simulink model "GroundSourceHX_oldGfunction"  (R2018b)
settings: Solver=ode23t  StartTime=0.0  StopTime=7*24*3600  RelTol=1e-3
values from neighbouring files (symbols this model uses):
  Ad = zeros(DimAxi/2,DimAxi/2)    [parameter_CARNOTews.m]
  Ad0 = zeros(DimAxi/2,DimAxi/2)    [parameter_CARNOTews.m]
  Ar = a    [parameter_CARNOTews.m]
  Au = zeros(DimAxi/2,DimAxi/2)    [parameter_CARNOTews.m]
  Au0 = zeros(DimAxi/2,DimAxi/2)    [parameter_CARNOTews.m]
  Bd = zeros(DimAxi/2,DimAxi/2+1)    [parameter_CARNOTews.m]
  Bd0 = zeros(DimAxi/2,DimAxi/2+1)    [parameter_CARNOTews.m]
  Br = b    (= 0.718333333333)    [parameter_CARNOTews.m]
  Bu = zeros(DimAxi/2,DimAxi/2+1)    [parameter_CARNOTews.m]
  Bu0 = zeros(DimAxi/2,DimAxi/2+1)    [parameter_CARNOTews.m]
  c1 = zeros(DimAxi/2,Dim1)    [parameter_CARNOTews.m]
  c33 = zeros(DimAxi,DimAxi/2)    [parameter_CARNOTews.m]
  c4 = c41    [parameter_CARNOTews.m]
  Cd = eye(DimAxi/2)    [parameter_CARNOTews.m]
  Cdl = Cdl'    [parameter_CARNOTews.m]
  Cr = eye((DimRad-2)*DimAxi/2)    [parameter_CARNOTews.m]
  Cu = Cd    [parameter_CARNOTews.m]
  Dd = zeros(DimAxi/2,DimAxi/2+1)    [parameter_CARNOTews.m]
  Dl = Sondelaenge/DimAxi*2    (= 50)    [parameter_CARNOTews.m]
  Dr = zeros((DimRad-2)*DimAxi/2,DimAxi)    [parameter_CARNOTews.m]
  Du = zeros(DimAxi/2,DimAxi/2+1)    [parameter_CARNOTews.m]
  gfunction = zeros(length(t_Trichter),length(r_Trichter))    [parameter_CARNOTews.m]
  L1 = 1/R1    [parameter_CARNOTews.m]
  Rechenradius = rm    (= 5)    [parameter_CARNOTews.m]
  T_null = TEarth0(end,:)'    [parameter_CARNOTews.m]
  t_start = 50*8560*3600    (= 1540800000)    [parameter_CARNOTews.m]
  Tdown_0 = Tearth_anf(:,1)    [parameter_CARNOTews.m]
  Tearth_anf = TEarth0(1:end-1,:)    [parameter_CARNOTews.m]
  Ts_Trichter = 7*24*3600    (= 604800)    [parameter_CARNOTews.m]
  Tup_0 = flipud(Tdown_0)    [parameter_CARNOTews.m]
undefined symbols (not defined in the file or in its folder): DiameterLastPiece, Temperature
libraries: carnot x3
settings Model: SimulationMode=accelerator  Creator=goettsche  LastModifiedBy=drhf
settings DataIOCC: SaveOutput=off  SaveTime=off

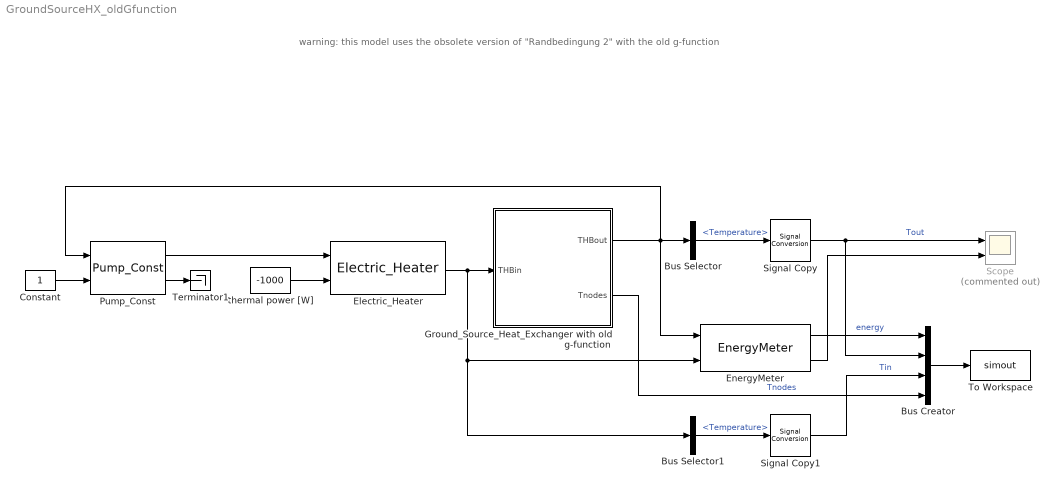
== system GroundSourceHX_oldGfunction ==
  note: warning: this model uses the obsolete version of "Randbedingung 2" with the old g-function
  Bus Creator : BusCreator  Inputs=4
  Bus Selector : BusSelector  OutputSignals=Temperature
  Bus Selector1 : BusSelector  OutputSignals=Temperature
  Constant : Constant
  Electric_Heater : carnot/Source/Boiler/Electric_Heater
      settings: SourceProductName=Carnot
  EnergyMeter : carnot/Control/EnergyMeter
      settings: SourceProductName=Carnot
  Ground_Source_Heat_Exchanger with old g-function : Subsystem  mask(ground source heat exchanger){Jahresmitteltemp_C=10, TGrad=0.025, lambdaErde=2.3, cpErde=800, rhoErde=2500, lambdaFill=2.1, cpFill=2500, rhoFill=800, Sondelaenge=50, B=10, Sondendurchmesser=0.03, Bohrdurchmesser=0.2, sondenfall=1 probe, np=1, DimVert=5, DimRad=5, Gitterfaktor=2.5, LastYear=20}
      mask prompts: Jahresmitteltemp_C "Average annual outdoor temperature  in °C"; TGrad "Temperature gradient in K/m, typical 0.025..0.04"; lambdaErde "Thermal conductivity ground in W/m/K"; cpErde "Heat capacity of the ground in J/kg/K"; rhoErde "Denstiy of the ground in kg/m³"; lambdaFill "Thermal conductivity filling in W/m/K"; cpFill "Heat capacity of the filling in J/kg/K"; rhoFill "Denstiy of the filling in kg/m³"; Sondelaenge "H: Length of earth probe in m"; B "B: probe distance in m"; Sondendurchmesser "Diameter of tube in m"; Bohrdurchmesser "Diameter of drilled hole in m"; sondenfall "Field geometry"; np "Number of parallel tubes"; DimVert "No. of vertical nodes (typical 5, minimum 2)"; DimRad "No. of horizontal (radial) nodes (typical 10, minimum 3)"; Gitterfaktor "grid factor (typical 2.5)"; LastYear "Last year of calculation (>= 1, set to 50 for steady state)"
      mask help:
      | The CARNOT EWS model is a transient model for dynamic simulation of borehole heat exchangers or so-called vertical ground heat exchangers. The model is based on the equations described by [Huber97] and has been implemented using the state space model of Matlab/Simulink [Bianchi06].
      | Bianchi M. A., Adaptive modellbasierte prädiktive Regelung einer Kleinwärmepumenanlage Diss. ETH Zuerich, No. 16892, 2006
      | Huber A, Schuler O., Berechnungsmodul für Erdwärmesonden (EWS). ENET Bericht Nr. 9658807-1, 1997
      mask init:
      | startfall = 2;
      | DimAxi = max(DimVert*2,4);
      | DimRad = max(DimRad,3);
      | 
      | [Ad,Bd,Cd,Dd, Au,Bu,Cu,Du, Ad0,Bd0, Au0,Bu0, ...
      |     Ar,Br,Cr,Dr, Cdl, c1, c3, c31, c33, c4, c41, c5, c6, ...
      |     L1, L2, L10, L20, Dl, Rechenradius, ...
      |     Tearth_anf, T_null, teta_fluid_ini, Tdown_0, Tup_0, ...
      |     Ts_Trichter, t_Trichter, r_Trichter, gfunction, t_start ...
      |     ] = ...
      |     CarnotCallbacks_EWS(startfall, LastYear, np, ...
      |     Jahresmitteltemp_C, TGrad, ...
      |     lambdaErde, rhoErde, cpErde, ...
      |     lambdaFill, cpFill, rhoFill, ...
      |     B, Sondelaenge, Sondendurchmesser, Bohrdurchmesser, ...
      |     DimAxi, DimRad, Gitterfaktor, sondenfall);
      | 
      | 
      | % % Sets the parameters for the model
      | % % ***********************************************************************
      | % % This file is part of the CARNOT Blockset.
      | % %   CARNOT is free software: you can redistribute it and/or modify
      | % %   it under the terms of the GNU Lesser General Public License as published by
      | % %   the Free Software Foundation, either version 3 of the License, or
      | % %   (at your option) any later version.
      | % %   CARNOT is distributed in the hope that it will be useful,
      | % %   but WITHOUT ANY WARRANTY; without even the implied warranty of
      | % %   MERCHANTABILITY or FITNESS FOR A PARTICULAR PURPOSE.  See the
      | % %   GNU Lesser General Public License for more details.
      | % %   You should have received a copy (copying_lesser.txt) of the 
      | % %   GNU Lesser General Public License along with CARNOT.  
      | % %   If not, see <http://www.gnu.org/licenses/>.
      | % %  
      | % % **********************************************************************
      | % % author list:      fab -> Fabian Ochs
      | % %                   hf  -> Bernd Hafner
      | % %
      | % % version: CarnotVersion.MajorVersionOfFunction.SubversionOfFunction
      | % %
      | % % Version  Author  Changes                                     Date
      | % % 5.1.0    fab     created, based on Diss. Bianchi ETH Zurich  01dec2012
      | % % 5.1.1    hf      adapted to carnot input and output struct.  04mar2013 
      | % %
      | % % Copyright (c) 2012 TU Insbruck, Fabian Ochs
      | % 
      | % startfall = 2; % 2: g-function
      | % mdot = 0.5;
      | % teta_in = 1;
      | % Massenstrom = mdot/np;
      | % Qdot0 = 5000;
      | % t_start = 50*8560*3600;
      | % 
      | % % Geometry
      | % Dicke_Sondenrohr = 0.003;
      | % lambda_Sondenrohr = 0.48;
      | % Bu = .1293;
      | % 
      | % % Ground Properties
      | % aErde = lambdaErde/(rhoErde*cpErde);
      | % 
      | % % Fluid
      | % teta_m = 2; 
      | % p0 = 1E5;
      | % fluid = 5;
      | % mix = 0.25;
      | % 
      | % Jahresmitteltemp=Jahresmitteltemp_C + 273.15;
      | % Bodenerwaermung=1;                          % 0°C
      | % Bodentemp=Jahresmitteltemp+Bodenerwaermung; % K
      | % 
      | % % Calculation
      | % lambdaSole=thermal_conductivity(teta_m,p0,fluid,mix);%W/(m K)
      | % cpSole=heat_capacity(teta_m,p0,fluid,mix);                                % J/Kg*K
      | % rhoSole=density(teta_m,p0,fluid,mix);%kg/m^3
      | % vSole=kinematic_viscosity(teta_m,p0,fluid,mix);                             % m2/s
      | % 
      | % Pr=vSole*rhoSole*cpSole/lambdaSole;
      | % rb = Bohrdurchmesser/2;
      | % rm = B/2;
      | % Rechenradius = rm;
      | % Dl=Sondelaenge/DimAxi*2;    
      | % 
      | % rs=Sondendurchmesser/2;
      | % r0 = rs-Dicke_Sondenrohr; % Innenradius
      | % r1=Bohrdurchmesser/2;
      | % r2=r1+(Rechenradius-r1)*(1-Gitterfaktor)/(1-Gitterfaktor^(DimRad-1))*Gitterfaktor^0;
      | % 
      | % rz1=((r1^2+r0^2)/2)^0.5;
      | % rz2=((r2^2+r1^2)/2)^0.5;
      | % 
      | % mcpSole=2*cpSole*rhoSole*pi*Dl*(Sondendurchmesser/2)^2;
      | % Di = Sondendurchmesser - 2 * Dicke_Sondenrohr;
      | % Geschw_Sole= Massenstrom/rhoSole/(Di/2)^2/pi/2; % 2: double U
      | % 
      | % Vdot = Massenstrom/rhoSole;
      | % A_p = (Di/2)^2/pi/2;
      | % 
      | % Re=Geschw_Sole*Di/vSole;
      | % Druckverlust= 1/(1.82*log10(Re)-1.64)^2;
      | % K1=1+27.2*Druckverlust/8;
      | % K1_o=1.106886;
      | % K2=11.7+1.8*Pr^(-1.3);
      | % Druckverlust_o=0.031437;
      | % St_o= Druckverlust_o/8/(K1_o+K2*(Druckverlust_o/8)^0.5*(Pr^(2/3)-1));
      | % Nu_o=St_o*10000*Pr;
      | % St= Druckverlust/8/(K1+K2*(Druckverlust/8)^0.5*(Pr^(2/3)-1));
      | % 
      | % % acc. Hellström    
      | % b = Bu/(2*r1);
      | % b_max = 1-rs/r1;
      | % b_min = rs/r1;
      | % sigma = (lambdaFill-lambdaErde)/(lambdaErde+lambdaFill);
      | % A = pi*r0^2;
      | % vs = Massenstrom/2/rhoSole/A;
      | % zeta = 1/((1.82*log10(Re)-1.64)^2);
      | % K1 = 1+27.2*zeta/8;
      | % K2 = 11.7+1.8*Pr^(-1/3); 
      | % R_s = 1/(2*pi*lambda_Sondenrohr)*log(rs/r0);
      | %     
      | % Nu_turbulent=St*Re*Pr;        
      | % Nu_laminar=4.36;
      | % 
      | % if Re>=10000,
      | %     Nu =(zeta/8)*Re*Pr/(K1+K2*(zeta/8)^.5*(Pr^(2/3)-1));
      | % elseif Re<10000 && Re>2300
      | %     Nu = Nu_laminar*exp(log(Nu_o/Nu_laminar)*log(Re/2300)/log(10000/2300));
      | % elseif Re<=2300,
      | %     Nu=Nu_laminar;        
      | % end
      | %     
      | % alpha = Nu*lambdaSole/(2*r0);
      | % alpha_eff = (1/alpha+r0/lambda_Sondenrohr*log(rs/r0))^-1;
      | % alpha0 = lambdaSole/(Di/2*(1-0.5^0.5));
      | % alpha0_eff = (1/alpha0+r0/lambda_Sondenrohr*log(rs/r0))^-1;
      | % 
      | % R_a = 1/(8*pi*alpha*r0);
      | % beta = lambdaFill*(1/(r0*alpha)+1/lambda_Sondenrohr*log(rs/r0));
      | % 
      | % R1_EWS=0.25*(1/(2*pi*alpha_eff*r0*Dl)+1/(2*pi*lambdaFill*Dl)*log((r1-rz1)/r0));
      | % R2_EWS=1/(2*pi*Dl)*(1/lambdaFill*log(r1/rz1)+1/lambdaErde*log(rz2/r1));        
      | % R10_EWS=0.25*(1/(2*pi*alpha0_eff*r0*Dl)+1/(2*pi*lambdaFill*Dl)*log((r1-rz1)/r0));
      | % R20_EWS=1/(2*pi*Dl)*(1/lambdaFill*log(r1/rz1)+1/lambdaErde*log(rz2/r1));        
      | % 
      | % Ra = 1/(pi*lambdaFill)*(log((2^.5*b*r1)/r0)-1/2*log((2*b*r1)/r0)-1/2*sigma*log((1-b^4)/(1+b^4)))+(1/(2*pi*r0*alpha))+R_s;
      | % Rb = (1/(8*pi*lambdaFill))*(beta+log(r1/r0)+log(r1/Bu)+sigma*log(r1^4/(r1^4-Bu^4/16))-(r0^2/Bu^2*(1-sigma*(Bu^474)/(r1^4-Bu^4/16)^2))/((1+beta)/(1-beta)+r0^2/Bu^2*(1+sigma*Bu^4*r1^4/(r1^4-Bu^4/16)^2)));
      | % Ra0 = 1/(pi*lambdaFill)*(log((2^.5*b*r1)/r0)-1/2*log((2*b*r1)/r0)-1/2*sigma*log((1-b^4)/(1+b^4)))+(1/(2*pi*r0*alpha0))+R_s;
      | % Rb0 = (1/(8*pi*lambdaFill))*(beta+log(r1/r0)+log(r1/Bu)+sigma*log(r1^4/(r1^4-Bu^4/16))-(r0^2/Bu^2*(1-sigma*(Bu^474)/(r1^4-Bu^4/16)^2))/((1+beta)/(1-beta)+r0^2/Bu^2*(1+sigma*Bu^4*r1^4/(r1^4-Bu^4/16)^2)));
      | % 
      | % if Ra < 4 * Rb
      | %     R1 = Ra/(4*Dl);
      | %     R2 = (Rb-Ra/4)/Dl+(2*pi*Dl*lambdaErde)^-1*log(rz2/r1);
      | %     R10 = Ra0/(4*Dl);
      | %     R20 = (Rb0-Ra0/4)/Dl+(2*pi*Dl*lambdaErde)^-1*log(rz2/r1);        
      | % else
      | %     R1 = R1_EWS;
      | %     R2 = R2_EWS;
      | %     R10 = R10_EWS;
      | %     R20 = R20_EWS;
      | % end
      | %     
      | % % temperaturverlauf axialer richtung
      | % L0=cpSole*Massenstrom;      % konstant
      | % L00 = 0.0;
      | % L1=1/R1;
      | % L2=1/R2;
      | % L10=1/R10;
      | % L20=1/R20;
      | % 
      | % % matrizen Ad,Bd,Cd,Dd für Tdown
      | % Ad=zeros(DimAxi/2,DimAxi/2);
      | % Ad0=zeros(DimAxi/2,DimAxi/2);
      | % for h=1:DimAxi/2,
      | %     Ad(h,h)=-(L0/(mcpSole)+L1/(2*mcpSole));
      | %     Ad0(h,h)=-(L00/(mcpSole)+L10/(2*mcpSole));
      | % end
      | %   
      | % for h=1:DimAxi/2-1,
      | %     Ad(h+1,h)=L0/(mcpSole);
      | %     Ad0(h+1,h)=L00/(mcpSole);
      | % end
      | % 
      | % Bd=zeros(DimAxi/2,DimAxi/2+1);
      | % Bd0=zeros(DimAxi/2,DimAxi/2+1);
      | % Bd(1,1)=L0/(mcpSole);
      | % Bd0(1,1)=L00/(mcpSole);
      | % 
      | % for h=1:DimAxi/2,
      | %     Bd(h,h+1)=L1/(2*mcpSole);
      | %     Bd0(h,h+1)=L10/(2*mcpSole);
      | % end
      | % 
      | % Cd=eye(DimAxi/2);
      | % Dd=zeros(DimAxi/2,DimAxi/2+1);
      | % 
      | % % matrizen Au,Bu,Cu,Du für Tup
      | % Au=zeros(DimAxi/2,DimAxi/2);
      | % Au0=zeros(DimAxi/2,DimAxi/2);
      | % for h=1:DimAxi/2,
      | %     Au(h,h)=-(L0/(mcpSole)+L1/(2*mcpSole));
      | %     Au0(h,h)=-(L00/(mcpSole)+L10/(2*mcpSole));
      | % end
      | %   
      | % for h=1:DimAxi/2-1,
      | %     Au(h+1,h)=L0/(mcpSole);
      | %     Au0(h+1,h)=L00/(mcpSole);
      | % end
      | % 
      | % Bu=zeros(DimAxi/2,DimAxi/2+1);
      | % Bu0=zeros(DimAxi/2,DimAxi/2+1);
      | % Bu(1,1)=L0/(mcpSole);
      | % Bu0(1,1)=L00/(mcpSole);
      | % for h=1:DimAxi/2,
      | %     Bu(h,h+1)=L1/(2*mcpSole);
      | %     Bu0(h,h+1)=L10/(2*mcpSole);
      | % end
      | % 
      | % Cu=Cd;
      | % Du=zeros(DimAxi/2,DimAxi/2+1);
      | % 
      | % % berechnung von Tradial, von Luzi Valär
      | % Dim1=(DimRad-2)*DimAxi/2;
      | % r = zeros(1:DimRad);
      | % r(1)=Bohrdurchmesser/2;
      | % r(2)=r2;
      | % for h =3:DimRad,
      | %     r(h)=r(h-1)+(Rechenradius-r1)*(1-Gitterfaktor)/(1-Gitterfaktor^(DimRad-1))*Gitterfaktor^(h-2);
      | % end
      | %     
      | % rz = zeros(1:DimRad);
      | % rz(1)=((r(1)^2+r0^2)/2)^0.5;
      | % for h = 2:DimRad,
      | %     rz(h)=((r(h)^2+r(h-1)^2)/2)^0.5;
      | % end
      | % 
      | % L = zeros(1:DimRad);
      | % L(1)=L1; 
      | % L(2)=L2;
      | % for h = 3:DimRad-1,
      | %     L(h)=1/(1/(2*pi*Dl)*(1/lambdaErde*log(rz(h)/rz(h-1))));
      | % end
      | % L(DimRad)=1/(1/(2*pi*Dl)*(1/lambdaErde*log(r(DimRad)/rz(DimRad-1))));
      | % 
      | % 
      | % C = zeros(1:DimRad);
      | % C(1)=cpFill*rhoFill*pi*(r(1)^2-4*r0^2)*Dl;
      | % for h = 2:DimRad,
      | %     C(h)=cpErde*rhoErde*pi*(r(h)^2-r(h-1)^2)*Dl;
      | % end
      | % 
      | % 
      | % a=zeros(DimRad-2,DimRad-2);
      | % for h = 1:DimRad-2,
      | %     a(h,h)=(-L(h)-L(h+1))/C(h);
      | % end
      | % for h = 1:DimRad-3,
      | %     a(h,h+1)=L(h+1)/C(h);
      | %     a(h+1,h)=L(h+1)/C(h+1);
      | % end
      | % 
      | % b=zeros(DimRad-2,2);
      | %     b(1,1)=L(1)/C(1);
      | %     b(DimRad-2,2)=L(DimRad-1)/C(DimRad-2);
      | %     
      | % %%%%%%%%%%%%%%%%%%%%%%%%%%%%%%%%%%%%%%%%%%%%%%%%%%% 
      | %     
      | % Ar=a;
      | % Ar(DimRad-1:2*(DimRad-2),DimRad-1:2*(DimRad-2))=a;
      | %     
      | % for h=2:DimAxi/2-1,
      | %     Ar(h*(DimRad-2)+1:(h+1)*(DimRad-2),h*(DimRad-2)+1:(h+1)*(DimRad-2))=a;
      | % 
      | % end  
      | % 
      | % Br=b;
      | % 
      | % for h=1:DimAxi/2-1,
      | %     Br(h*(DimRad-2)+1:(h+1)*(DimRad-2),2*h+1:2*h+2)=b;   
      | % end
      | %     
      | % 
      | % Cr=eye((DimRad-2)*DimAxi/2);
      | % Dr=zeros((DimRad-2)*DimAxi/2,DimAxi);
      | % 
      | % % andere matrizen
      | % Cdl=zeros(DimAxi/2,1);
      | % Cdl(DimAxi/2,1)=1;
      | % Cdl=Cdl';
      | % 
      | % c1=zeros(DimAxi/2,Dim1);
      | % for h=1:DimAxi/2,
      | %     c1(1,1)=1;
      | %     c1(h,(h-1)*(DimRad-2)+1)=1;
      | % end
      | % 
      | % c31=zeros(1,DimAxi/2);
      | % c3(1,1)=1;
      | % for h=1:DimAxi/2-1,
      | %     c3(1+2*h,1+h)=1;
      | % end
      | % 
      | % c33=zeros(DimAxi,DimAxi/2);
      | % c33(1:DimAxi-1,1:DimAxi/2)=c3;
      | % 
      | % c41=zeros(1,DimAxi/2);
      | % c4=c41;
      | % c4(2:DimAxi,1:DimAxi/2)=c3;
      | % 
      | % 
      | % % randbedingungen für Tearth,DimRad
      | % % anfangsbedingungen für Tradial
      | % mu=linspace(0,Sondelaenge,DimAxi/2);
      | % T=(mu*TGrad+Bodentemp);
      | % Tearth_anf=T'*ones(1,DimRad-2);
      | % T_null=Tearth_anf(:,1);
      | % teta_fluid_ini = mean(T_null)-273.15;
      | % 
      | % % anfangsbedingungen für Tdown,Tup
      | % Tdown_0=Tearth_anf(:,1);
      | % Tup_0=flipud(Tdown_0);
      | % Tearth_anf=Tearth_anf';
      | % c5=ones(DimAxi/2,1);           
      | % 
      | % c6=zeros(DimRad-2,3*(DimRad-2));
      | % 
      | % for i=2:DimRad-2;
      | %     c6(1,DimRad-1)=1;
      | %     c6(i,DimRad+i-2)=1;
      | % end
      | % 
      | % %% RB
      | % Ts_Trichter=7*24*3600; % 7 (1 week according to Huber)
      | % Dr_Trichter=1;
      | % t_Trichter = linspace(Ts_Trichter,Ts_Trichter*5000,5000);
      | % r_Trichter = linspace(Dr_Trichter,Dr_Trichter*20,20);
      | % 
      | % % g-function
      | % xS = [-4 -2 0 2 3];
      | % if sondenfall == 1          % 1 Sonde
      | %     yS = [4.82 5.69 6.29 6.57 6.6];
      | % elseif sondenfall == 2      % 2 Sonden B/H = 0.1
      | %     yS = [4.99 6.37 7.62 8.06 8.08];
      | % elseif sondenfall == 3      % 2 Sonden B/H = 0.05
      | %     yS = [5.30 6.92 8.20 8.67 8.71];
      | % elseif sondenfall == 4      % 3x6 Sonden B/H = 0.1
      | %     yS = [5.00 9.15 16.40 19.75 20.05];
      | % elseif sondenfall == 5      % 5x10 Sonden B/H = 0.1
      | %     yS = [5.00 10.2 22.75 29.5 30.05];
      | % end
      | % 
      | % npol = 4;
      | % p = polyfit(xS,yS,npol);
      | % ts = Sondelaenge^2/(9*aErde);
      | % gfunction = zeros(length(t_Trichter),length(r_Trichter));
      | % Es = t_Trichter*9*aErde/Sondelaenge^2;
      | % 
      | % g = polyval(p,log(Es));
      | % 
      | % for ii = 1:length(r_Trichter)
      | %     gfunction(:,ii) = max(0,g - log(r_Trichter(ii)/Sondelaenge/0.0005)); % correction 21-09-2012
      | % end
      | % 
      | % % Startwerte
      | % qdot0 = Qdot0/Sondelaenge; 
      | % if startfall == 2
      | %     Es_start = t_start*9*aErde/Sondelaenge^2;
      | %     TEarth0 = zeros(size(Tearth_anf));
      | %     for ii = 1:DimAxi/2
      | %         for iii = 1:DimRad-1
      | %             g_start = polyval(p,log(Es_start));
      | %             TEarth0(iii,ii) = Bodentemp + mu(ii)*TGrad - qdot0/(DimAxi/2)*((g_start-log(rz(iii+1)/Sondelaenge/0.0005))/(2*pi*lambdaErde));
      | %         end
      | %     end    
      | % 
      | %     T_null = TEarth0(end,:)';
      | %     Tearth_anf = TEarth0(1:end-1,:);
      | % end
      mask Help: web(fullfile(path_carnot('help'),'Ground_Source_Heat_Exchanger.html'),'-helpbrowser')
      mask TypeOptions sondenfall: 1 probe | 2 probes B/H = 0.1 | 2 probes B/H = 0.05 | 3x6 probes B/H = 0.1 | 5x10 probes B/H = 0.1
      mask DialogControl ParameterTabVar0 Prompt: General
      mask DialogControl ParameterTabVar01 Prompt: Geometry
      mask DialogControl ParameterTabVar012 Prompt: Calculation
      mask Display: plot(0,10,100,90,[70,30],[80,80],[35,35,43,43,47,52,57,57,66,66,60,60,54,46,40,40,35],[84,87,87,20,13,13,21,87,87,84,84,20,10,10,20,84,84])
  Pump_Const : carnot/Hydraulics/Pump_Const  mdotmax=0.44  dia=0.02  p0=3e5  fluid_id=Water-Glycol Mix  mix=0.25  mix2=0  mix3=0  UA=3  mcp=4182  Tini=20  e0=10  e1=10  e2=-1
      settings: SourceProductName=Carnot
  Scope : Scope  Commented=on  NumInputPorts=2
  Signal Copy : SignalConversion  OverrideOpt=off
  Signal Copy1 : SignalConversion  OverrideOpt=off
  Terminator1 : Terminator
  To Workspace : ToWorkspace  VariableName=simout  SaveFormat=Timeseries  SampleTime=3600
  thermal power [W] : Constant  Value=-1000
  wires:
  Ground_Source_Heat_Exchanger with old g-function/1(THBout) -> Bus Selector/1, EnergyMeter/1, Pump_Const/1
  Bus Selector/1 -> Signal Copy/1  "<Temperature>"
  EnergyMeter/2 -> Scope/2
  Ground_Source_Heat_Exchanger with old g-function/2(Tnodes) -> Bus Creator/4  "Tnodes"
  Electric_Heater/1 -> Bus Selector1/1, EnergyMeter/2, Ground_Source_Heat_Exchanger with old g-function/1(THBin)
  thermal power [W]/1 -> Electric_Heater/2
  Pump_Const/1 -> Electric_Heater/1
  Constant/1 -> Pump_Const/2
  Pump_Const/2 -> Terminator1/1
  EnergyMeter/1 -> Bus Creator/1  "energy"
  Bus Creator/1 -> To Workspace/1
  Signal Copy/1 -> Bus Creator/2, Scope/1  "Tout"
  Bus Selector1/1 -> Signal Copy1/1  "<Temperature>"
  Signal Copy1/1 -> Bus Creator/3  "Tin"

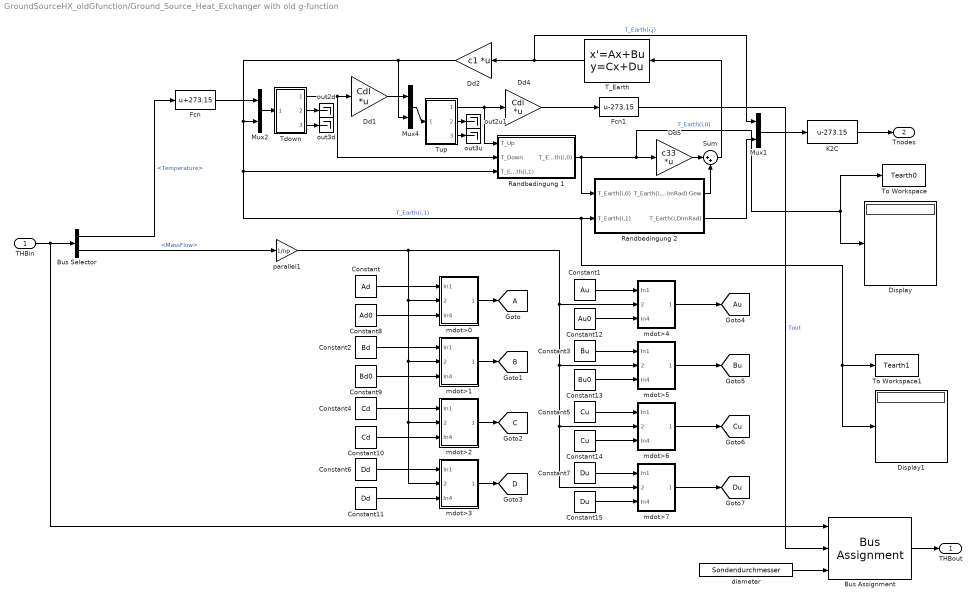
== system GroundSourceHX_oldGfunction/Ground_Source_Heat_Exchanger with old g-function ==
  THBin : Inport
  Bus Assignment : BusAssignment  AssignedSignals=Temperature,DiameterLastPiece
  Bus Selector : BusSelector  OutputSignals=Temperature,MassFlow
  Constant : Constant  Value=Ad
  Constant1 : Constant  Value=Au
  Constant10 : Constant  Value=Cd
  Constant11 : Constant  Value=Dd
  Constant12 : Constant  Value=Au0
  Constant13 : Constant  Value=Bu0
  Constant14 : Constant  Value=Cu
  Constant15 : Constant  Value=Du
  Constant2 : Constant  Value=Bd
  Constant3 : Constant  Value=Bu
  Constant4 : Constant  Value=Cd
  Constant5 : Constant  Value=Cu
  Constant6 : Constant  Value=Dd
  Constant7 : Constant  Value=Du
  Constant8 : Constant  Value=Ad0
  Constant9 : Constant  Value=Bd0
  Dd1 : Gain  Gain=Cdl  Multiplication=Matrix(K*u)  SaturateOnIntegerOverflow=on  OutDataTypeStr=Inherit: Same as input  ParamDataTypeStr=Inherit: Same as input
  Dd2 : Gain  Gain=c1  Multiplication=Matrix(K*u)  SaturateOnIntegerOverflow=on  OutDataTypeStr=Inherit: Same as input  ParamDataTypeStr=Inherit: Same as input
  Dd4 : Gain  Gain=Cdl  Multiplication=Matrix(K*u)  SaturateOnIntegerOverflow=on  OutDataTypeStr=Inherit: Same as input  ParamDataTypeStr=Inherit: Same as input
  Dd5 : Gain  Gain=c33  Multiplication=Matrix(K*u)  SaturateOnIntegerOverflow=on  OutDataTypeStr=Inherit: Same as input  ParamDataTypeStr=Inherit: Same as input
  Display : Display
  Display1 : Display
  Fcn : Fcn  Expr=u+273.15
  Fcn1 : Fcn  Expr=u-273.15
  K2C : Bias  Bias=-273.15
  Mux1 : Mux  Inputs=2
  Mux2 : Mux  Inputs=2
  Mux4 : Mux  Inputs=2
  Randbedingung 1 : Subsystem
  Randbedingung 2 : Subsystem
  Sum : Sum  Inputs=|++  SaturateOnIntegerOverflow=on  InputSameDT=on  OutDataTypeStr=Inherit: Same as first input
  T_Earth : StateSpace  A=Ar  B=Br  C=Cr  D=Dr  InitialCondition=Tearth_anf(:)
  Tdown : Subsystem
  To Workspace : ToWorkspace  VariableName=Tearth0  SampleTime=-1
      settings: MaxDataPoints=1
  To Workspace1 : ToWorkspace  VariableName=Tearth1  SampleTime=-1
      settings: MaxDataPoints=1
  Tup : Subsystem
  diameter : Constant  Value=Sondendurchmesser
  mdot>0 : Subsystem
  mdot>1 : Subsystem
  mdot>2 : Subsystem
  mdot>3 : Subsystem
  mdot>4 : Subsystem
  mdot>5 : Subsystem
  mdot>6 : Subsystem
  mdot>7 : Subsystem
  out2d : Terminator
  out2u1 : Terminator
  out3d : Terminator
  out3u : Terminator
  parallel1 : Gain  Gain=1/np
  THBout : Outport
  Tnodes : Outport  Port=2
  tag scope: A=global, Au=global, B=global, Bu=global, C=global, Cu=global, D=global, Du=global
  wires:
  K2C/1 -> Tnodes/1
  Bus Selector/1 -> Fcn/1  "<Temperature>"
  Bus Selector/2 -> parallel1/1  "<MassFlow>"
  Mux1/1 -> K2C/1
  parallel1/1 -> mdot>7/2(mdot), mdot>6/2(mdot), mdot>5/2(mdot), mdot>4/2(mdot), mdot>3/2(mdot), mdot>2/2(mdot), mdot>1/2(mdot), mdot>0/2(mdot)
  Constant12/1 -> mdot>4/3(In4)
  Constant13/1 -> mdot>5/3(In4)
  Constant14/1 -> mdot>6/3(In4)
  Constant15/1 -> mdot>7/3(In4)
  mdot>4/1(Out1) -> [Au]
  mdot>5/1(Out1) -> [Bu]
  mdot>6/1(Out1) -> [Cu]
  mdot>7/1(Out1) -> [Du]
  Constant7/1 -> mdot>7/1(In1)
  Constant5/1 -> mdot>6/1(In1)
  Constant3/1 -> mdot>5/1(In1)
  Constant1/1 -> mdot>4/1(In1)
  Constant6/1 -> mdot>3/1(In1)
  Constant11/1 -> mdot>3/3(In4)
  Constant10/1 -> mdot>2/3(In4)
  mdot>3/1(Out1) -> [D]
  Constant4/1 -> mdot>2/1(In1)
  mdot>2/1(Out1) -> [C]
  Constant9/1 -> mdot>1/3(In4)
  Constant2/1 -> mdot>1/1(In1)
  Constant/1 -> mdot>0/1(In1)
  mdot>1/1(Out1) -> [B]
  Constant8/1 -> mdot>0/3(In4)
  mdot>0/1(Out1) -> [A]
  Tup/2(Out2) -> out2u1/1
  Tdown/2(Out2) -> out2d/1
  Tup/3(Out3) -> out3u/1
  Tdown/3(Out3) -> out3d/1
  Tdown/1(Out1) -> Randbedingung 1/2(T_Down), Dd1/1
  Mux2/1 -> Tdown/1(In1)
  Mux4/1 -> Tup/1(In1)
  Dd1/1 -> Mux4/1
  T_Earth/1 -> Mux1/1, Dd2/1  "T_Earth(i,j)"
  Tup/1(Out1) -> Randbedingung 1/1(T_Up), Dd4/1
  Dd4/1 -> Fcn1/1
  Dd5/1 -> Sum/1
  Randbedingung 2/1(T_Earth(i,DimRad) Gew) -> Sum/2
  Sum/1 -> T_Earth/1
  Randbedingung 1/1(T_Earth(i,0)) -> To Workspace/1, Display/1, Dd5/1, Randbedingung 2/1(T_Earth(i,0))  "T_Earth(i,0)"
  Dd2/1 -> Mux4/2, To Workspace1/1, Display1/1, Randbedingung 2/2(T_Earth(i,1)), Randbedingung 1/3(T_Earth(i,1)), Mux2/2  "T_Earth(i,1)"
  Randbedingung 2/2(T_Earth(i,DimRad)) -> Mux1/2
  Fcn1/1 -> Bus Assignment/2  "Tout"
  Fcn/1 -> Mux2/1
  THBin/1 -> Bus Selector/1, Bus Assignment/1
  diameter/1 -> Bus Assignment/3
  Bus Assignment/1 -> THBout/1

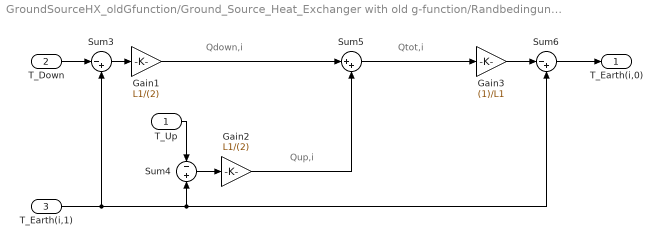
== system GroundSourceHX_oldGfunction/Ground_Source_Heat_Exchanger with old g-function/Randbedingung 1 ==
  note: Qdown,i
  note: Qup,i
  note: Qtot,i
  T_Up : Inport
  T_Down : Inport  Port=2
  T_Earth(i,1) : Inport  Port=3
  Gain1 : Gain  Gain=L1/(2)  SaturateOnIntegerOverflow=on  OutDataTypeStr=Inherit: Same as input  ParamDataTypeStr=Inherit: Same as input
  Gain2 : Gain  Gain=L1/(2)  SaturateOnIntegerOverflow=on  OutDataTypeStr=Inherit: Same as input  ParamDataTypeStr=Inherit: Same as input
  Gain3 : Gain  Gain=(1)/L1  SaturateOnIntegerOverflow=on  OutDataTypeStr=Inherit: Same as input  ParamDataTypeStr=Inherit: Same as input
  Sum3 : Sum  Inputs=|-+  SaturateOnIntegerOverflow=on  InputSameDT=on  OutDataTypeStr=Inherit: Same as first input
  Sum4 : Sum  Inputs=-+  SaturateOnIntegerOverflow=on  InputSameDT=on  OutDataTypeStr=Inherit: Same as first input
  Sum5 : Sum  Inputs=|++  SaturateOnIntegerOverflow=on  InputSameDT=on  OutDataTypeStr=Inherit: Same as first input
  Sum6 : Sum  Inputs=|-+  SaturateOnIntegerOverflow=on  InputSameDT=on  OutDataTypeStr=Inherit: Same as first input
  T_Earth(i,0) : Outport
  wires:
  Sum3/1 -> Gain1/1
  Sum4/1 -> Gain2/1
  Gain1/1 -> Sum5/1
  Gain2/1 -> Sum5/2
  Sum5/1 -> Gain3/1
  Gain3/1 -> Sum6/1
  T_Down/1 -> Sum3/1
  T_Up/1 -> Sum4/1
  T_Earth(i,1)/1 -> Sum3/2, Sum4/2, Sum6/2
  Sum6/1 -> T_Earth(i,0)/1

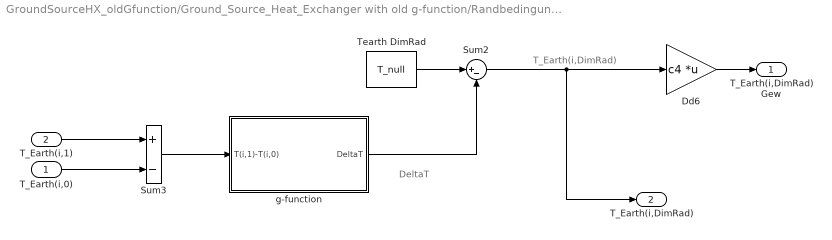
== system GroundSourceHX_oldGfunction/Ground_Source_Heat_Exchanger with old g-function/Randbedingung 2 ==
  note: T_Earth(i,DimRad)
  note: DeltaT
  T_Earth(i,0) : Inport
  T_Earth(i,1) : Inport  Port=2
  Dd6 : Gain  Gain=c4  Multiplication=Matrix(K*u)  SaturateOnIntegerOverflow=on  OutDataTypeStr=Inherit: Same as input  ParamDataTypeStr=Inherit: Same as input
  Sum2 : Sum  Inputs=|+-  SaturateOnIntegerOverflow=on  InputSameDT=on  OutDataTypeStr=Inherit: Same as first input
  Sum3 : Sum  Inputs=+-  SaturateOnIntegerOverflow=on  InputSameDT=on  OutDataTypeStr=Inherit: Same as first input
  Tearth DimRad : Constant  Value=T_null  VectorParams1D=off
  g-function : Subsystem
  T_Earth(i,DimRad) Gew : Outport
  T_Earth(i,DimRad) : Outport  Port=2
  wires:
  Sum2/1 -> Dd6/1, T_Earth(i,DimRad)/1
  Tearth DimRad/1 -> Sum2/1
  T_Earth(i,1)/1 -> Sum3/1
  T_Earth(i,0)/1 -> Sum3/2
  Dd6/1 -> T_Earth(i,DimRad) Gew/1
  Sum3/1 -> g-function/1(T(i,1)-T(i,0))
  g-function/1(DeltaT) -> Sum2/2

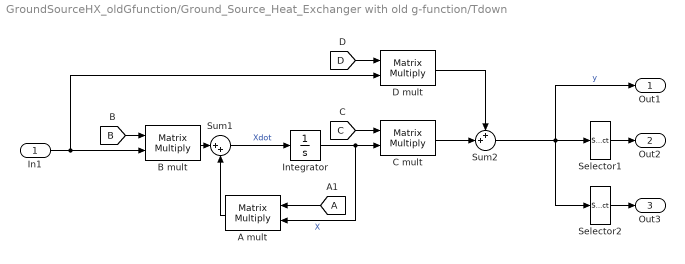
== system GroundSourceHX_oldGfunction/Ground_Source_Heat_Exchanger with old g-function/Tdown ==
  In1 : Inport
  A mult : Product  Multiplication=Matrix(*)  RndMeth=Zero
  B mult : Product  Multiplication=Matrix(*)  RndMeth=Zero
  C mult : Product  Multiplication=Matrix(*)  RndMeth=Zero
  D mult : Product  Multiplication=Matrix(*)  RndMeth=Zero
  Integrator : Integrator  InitialCondition=Tdown_0
  Selector1 : Selector  InputPortWidth=DimAxi/2  IndexOptions=Index vector (dialog)  Indices=1  OutputSizes=1
  Selector2 : Selector  InputPortWidth=DimAxi/2  IndexOptions=Index vector (dialog)  Indices=2  OutputSizes=1
  Sum1 : Sum  Inputs=|++
  Sum2 : Sum  Inputs=++|
  Out1 : Outport
  Out2 : Outport  Port=2
  Out3 : Outport  Port=3
  wires:
  Selector2/1 -> Out3/1
  Selector1/1 -> Out2/1
  [D] -> D mult/1
  [C] -> C mult/1
  [A] -> A mult/1
  [B] -> B mult/1
  A mult/1 -> Sum1/2
  Integrator/1 -> C mult/2, A mult/2  "X"
  Sum1/1 -> Integrator/1  "Xdot"
  B mult/1 -> Sum1/1
  C mult/1 -> Sum2/2
  D mult/1 -> Sum2/1
  In1/1 -> D mult/2, B mult/2
  Sum2/1 -> Out1/1, Selector1/1, Selector2/1  "y"

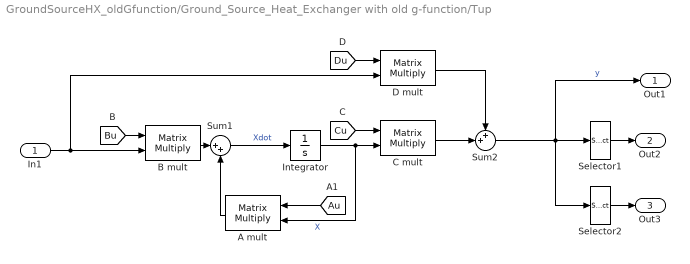
== system GroundSourceHX_oldGfunction/Ground_Source_Heat_Exchanger with old g-function/Tup ==
  In1 : Inport
  A mult : Product  Multiplication=Matrix(*)  RndMeth=Zero
  B mult : Product  Multiplication=Matrix(*)  RndMeth=Zero
  C mult : Product  Multiplication=Matrix(*)  RndMeth=Zero
  D mult : Product  Multiplication=Matrix(*)  RndMeth=Zero
  Integrator : Integrator  InitialCondition=Tup_0
  Selector1 : Selector  InputPortWidth=DimAxi/2  IndexOptions=Index vector (dialog)  Indices=1  OutputSizes=1
  Selector2 : Selector  InputPortWidth=DimAxi/2  IndexOptions=Index vector (dialog)  Indices=2  OutputSizes=1
  Sum1 : Sum  Inputs=|++
  Sum2 : Sum  Inputs=++|
  Out1 : Outport
  Out2 : Outport  Port=2
  Out3 : Outport  Port=3
  wires:
  Selector2/1 -> Out3/1
  Selector1/1 -> Out2/1
  [Du] -> D mult/1
  [Cu] -> C mult/1
  [Au] -> A mult/1
  [Bu] -> B mult/1
  A mult/1 -> Sum1/2
  Integrator/1 -> C mult/2, A mult/2  "X"
  Sum1/1 -> Integrator/1  "Xdot"
  B mult/1 -> Sum1/1
  C mult/1 -> Sum2/2
  D mult/1 -> Sum2/1
  In1/1 -> D mult/2, B mult/2
  Sum2/1 -> Out1/1, Selector1/1, Selector2/1  "y"

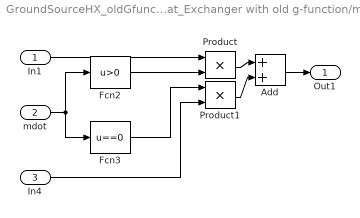
== system GroundSourceHX_oldGfunction/Ground_Source_Heat_Exchanger with old g-function/mdot>0 ==
  In1 : Inport
  mdot : Inport  Port=2
  In4 : Inport  Port=3
  Add : Sum
  Fcn2 : Fcn  Expr=u>0
  Fcn3 : Fcn  Expr=u==0
  Product : Product  RndMeth=Zero
  Product1 : Product  RndMeth=Zero
  Out1 : Outport
  wires:
  Fcn3/1 -> Product1/1
  Fcn2/1 -> Product/2
  mdot/1 -> Fcn3/1, Fcn2/1
  In4/1 -> Product1/2
  Add/1 -> Out1/1
  In1/1 -> Product/1
  Product1/1 -> Add/2
  Product/1 -> Add/1

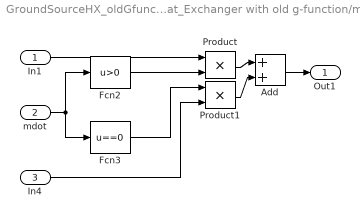
== system GroundSourceHX_oldGfunction/Ground_Source_Heat_Exchanger with old g-function/mdot>1 ==
  In1 : Inport
  mdot : Inport  Port=2
  In4 : Inport  Port=3
  Add : Sum
  Fcn2 : Fcn  Expr=u>0
  Fcn3 : Fcn  Expr=u==0
  Product : Product  RndMeth=Zero
  Product1 : Product  RndMeth=Zero
  Out1 : Outport
  wires:
  Fcn3/1 -> Product1/1
  Fcn2/1 -> Product/2
  mdot/1 -> Fcn3/1, Fcn2/1
  In4/1 -> Product1/2
  Add/1 -> Out1/1
  In1/1 -> Product/1
  Product1/1 -> Add/2
  Product/1 -> Add/1

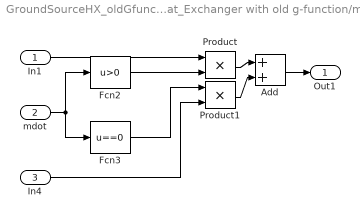
== system GroundSourceHX_oldGfunction/Ground_Source_Heat_Exchanger with old g-function/mdot>2 ==
  In1 : Inport
  mdot : Inport  Port=2
  In4 : Inport  Port=3
  Add : Sum
  Fcn2 : Fcn  Expr=u>0
  Fcn3 : Fcn  Expr=u==0
  Product : Product  RndMeth=Zero
  Product1 : Product  RndMeth=Zero
  Out1 : Outport
  wires:
  Fcn3/1 -> Product1/1
  Fcn2/1 -> Product/2
  mdot/1 -> Fcn3/1, Fcn2/1
  In4/1 -> Product1/2
  Add/1 -> Out1/1
  In1/1 -> Product/1
  Product1/1 -> Add/2
  Product/1 -> Add/1

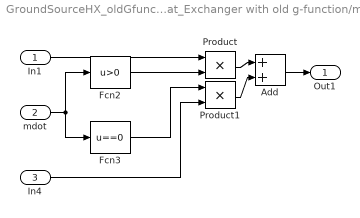
== system GroundSourceHX_oldGfunction/Ground_Source_Heat_Exchanger with old g-function/mdot>3 ==
  In1 : Inport
  mdot : Inport  Port=2
  In4 : Inport  Port=3
  Add : Sum
  Fcn2 : Fcn  Expr=u>0
  Fcn3 : Fcn  Expr=u==0
  Product : Product  RndMeth=Zero
  Product1 : Product  RndMeth=Zero
  Out1 : Outport
  wires:
  Fcn3/1 -> Product1/1
  Fcn2/1 -> Product/2
  mdot/1 -> Fcn3/1, Fcn2/1
  In4/1 -> Product1/2
  Add/1 -> Out1/1
  In1/1 -> Product/1
  Product1/1 -> Add/2
  Product/1 -> Add/1

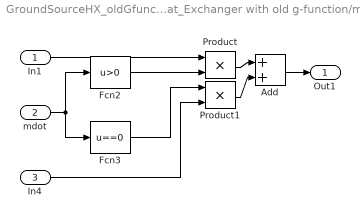
== system GroundSourceHX_oldGfunction/Ground_Source_Heat_Exchanger with old g-function/mdot>4 ==
  In1 : Inport
  mdot : Inport  Port=2
  In4 : Inport  Port=3
  Add : Sum
  Fcn2 : Fcn  Expr=u>0
  Fcn3 : Fcn  Expr=u==0
  Product : Product  RndMeth=Zero
  Product1 : Product  RndMeth=Zero
  Out1 : Outport
  wires:
  Fcn3/1 -> Product1/1
  Fcn2/1 -> Product/2
  mdot/1 -> Fcn3/1, Fcn2/1
  In4/1 -> Product1/2
  Add/1 -> Out1/1
  In1/1 -> Product/1
  Product1/1 -> Add/2
  Product/1 -> Add/1

== system GroundSourceHX_oldGfunction/Ground_Source_Heat_Exchanger with old g-function/mdot>5 ==
  In1 : Inport
  mdot : Inport  Port=2
  In4 : Inport  Port=3
  Add : Sum
  Fcn2 : Fcn  Expr=u>0
  Fcn3 : Fcn  Expr=u==0
  Product : Product  RndMeth=Zero
  Product1 : Product  RndMeth=Zero
  Out1 : Outport
  wires:
  Fcn3/1 -> Product1/1
  Fcn2/1 -> Product/2
  mdot/1 -> Fcn3/1, Fcn2/1
  In4/1 -> Product1/2
  Add/1 -> Out1/1
  In1/1 -> Product/1
  Product1/1 -> Add/2
  Product/1 -> Add/1

== system GroundSourceHX_oldGfunction/Ground_Source_Heat_Exchanger with old g-function/mdot>6 ==
  In1 : Inport
  mdot : Inport  Port=2
  In4 : Inport  Port=3
  Add : Sum
  Fcn2 : Fcn  Expr=u>0
  Fcn3 : Fcn  Expr=u==0
  Product : Product  RndMeth=Zero
  Product1 : Product  RndMeth=Zero
  Out1 : Outport
  wires:
  Fcn3/1 -> Product1/1
  Fcn2/1 -> Product/2
  mdot/1 -> Fcn3/1, Fcn2/1
  In4/1 -> Product1/2
  Add/1 -> Out1/1
  In1/1 -> Product/1
  Product1/1 -> Add/2
  Product/1 -> Add/1

== system GroundSourceHX_oldGfunction/Ground_Source_Heat_Exchanger with old g-function/mdot>7 ==
  In1 : Inport
  mdot : Inport  Port=2
  In4 : Inport  Port=3
  Add : Sum
  Fcn2 : Fcn  Expr=u>0
  Fcn3 : Fcn  Expr=u==0
  Product : Product  RndMeth=Zero
  Product1 : Product  RndMeth=Zero
  Out1 : Outport
  wires:
  Fcn3/1 -> Product1/1
  Fcn2/1 -> Product/2
  mdot/1 -> Fcn3/1, Fcn2/1
  In4/1 -> Product1/2
  Add/1 -> Out1/1
  In1/1 -> Product/1
  Product1/1 -> Add/2
  Product/1 -> Add/1

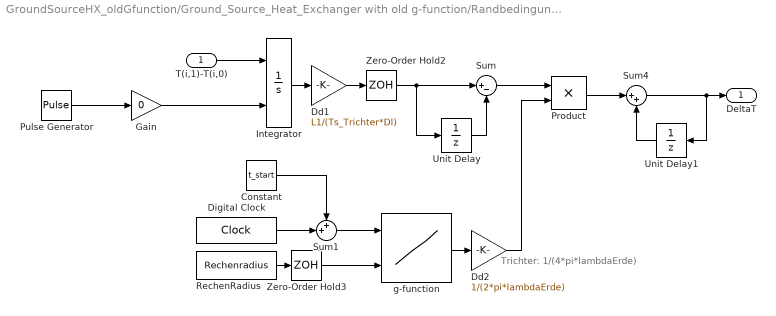
== system GroundSourceHX_oldGfunction/Ground_Source_Heat_Exchanger with old g-function/Randbedingung 2/g-function ==
  note: Trichter: 1/(4*pi*lambdaErde)
  T(i,1)-T(i,0) : Inport
  Constant : Constant  Value=t_start
  Dd1 : Gain  Gain=L1/(Ts_Trichter*Dl)  SaturateOnIntegerOverflow=on  OutDataTypeStr=Inherit: Same as input  ParamDataTypeStr=Inherit: Same as input
  Dd2 : Gain  Gain=1/(2*pi*lambdaErde)  SaturateOnIntegerOverflow=on  OutDataTypeStr=Inherit: Same as input  ParamDataTypeStr=Inherit: Same as input
  Digital Clock : DigitalClock
  Gain : Gain  Gain=0
  Integrator : Integrator  ExternalReset=rising
  Product : Product  SaturateOnIntegerOverflow=on  RndMeth=Zero  InputSameDT=on  OutDataTypeStr=Inherit: Same as first input
  Pulse Generator : DiscretePulseGenerator  PulseType=Time based  Period=Ts_Trichter  PulseWidth=50  PhaseDelay=300
  RechenRadius : Constant  Value=Rechenradius  VectorParams1D=off
  Sum : Sum  Inputs=|+-  SaturateOnIntegerOverflow=on  InputSameDT=on  OutDataTypeStr=Inherit: Same as first input
  Sum1 : Sum  Inputs=++|  SaturateOnIntegerOverflow=on  InputSameDT=on  OutDataTypeStr=Inherit: Same as first input
  Sum4 : Sum  Inputs=|++  SaturateOnIntegerOverflow=on  InputSameDT=on  OutDataTypeStr=Inherit: Same as first input
  Unit Delay : UnitDelay
  Unit Delay1 : UnitDelay
  Zero-Order Hold2 : ZeroOrderHold
  Zero-Order Hold3 : ZeroOrderHold
  g-function : Lookup2D  RowIndex=t_Trichter  ColumnIndex=r_Trichter  Table=gfunction  SaturateOnIntegerOverflow=on  InputSameDT=on
  DeltaT : Outport
  wires:
  Constant/1 -> Sum1/1
  Sum1/1 -> g-function/1
  Digital Clock/1 -> Sum1/2
  Pulse Generator/1 -> Gain/1
  Integrator/1 -> Dd1/1
  Dd1/1 -> Zero-Order Hold2/1
  Unit Delay/1 -> Sum/2
  Sum/1 -> Product/1
  g-function/1 -> Dd2/1
  RechenRadius/1 -> Zero-Order Hold3/1
  Product/1 -> Sum4/1
  Dd2/1 -> Product/2
  Unit Delay1/1 -> Sum4/2
  Sum4/1 -> Unit Delay1/1, DeltaT/1
  Zero-Order Hold3/1 -> g-function/2
  Zero-Order Hold2/1 -> Unit Delay/1, Sum/1
  T(i,1)-T(i,0)/1 -> Integrator/1
  Gain/1 -> Integrator/2
